simulink model "CH3_1"  (Simulink 5.0)
settings: Solver=ode15s  SolverMode=SingleTasking  StartTime=0.0  StopTime=3/60  RelTol=1e-3  AbsTol=1e-3
libraries: powerlib_extras x3
Description:
  | 高苑科技大學 電機系
  | 電力電子實驗室
settings Model: Creator=徐瑞隆老師  LastModifiedBy=ELECTRONIC  ExtModeTrigMode=oneshot  ExtModeArmWhenConnect=off  MaxOrder=4  LimitDataPoints=off  BlockReductionOpt=off  BooleanDataType=off  RTWTemplateMakefile=grt_unix.tmf

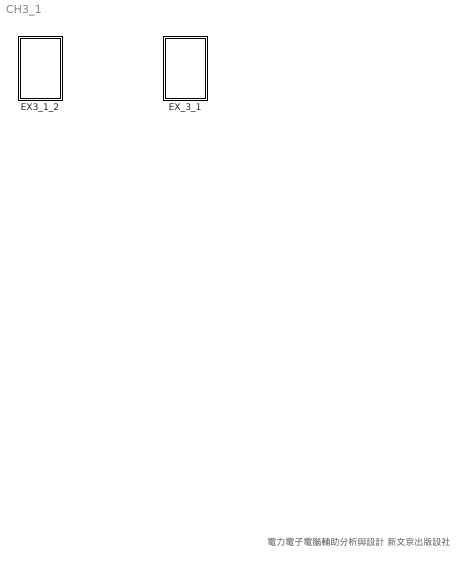
== system CH3_1 ==
  note: 電力電子電腦輔助分析與設計 新文京出版設社
  EX3_1_2 : Subsystem
  EX_3_1 : Subsystem

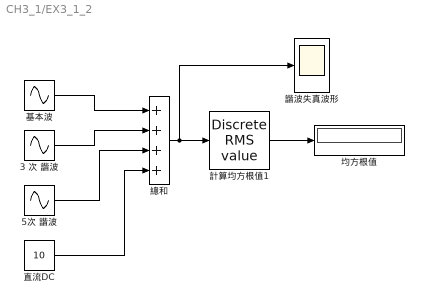
== system CH3_1/EX3_1_2 ==
  "3 次 諧波 " : Sin  Amplitude=8  Frequency=2*pi*180  Phase=1  SampleTime=0
  5次 諧波 : Sin  Amplitude=2  Frequency=2*pi*300  SampleTime=0
  "均方根值 " : Display
  直流DC : Constant  Value=10
  計算均方根值1 : powerlib_extras/Discrete Measurements/Discrete  RMS value  Freq=60  Mag_Init=0  Ts=50e-6
  基本波 : Sin  Amplitude=8  Frequency=2*pi*60  SampleTime=0
  諧波失真波形 : Scope
      settings: TimeRange=0.1  YMin=-3.5  YMax=3.5  SaveName=psb1phPWM3_str1  MaxDataPoints=50000
  總和 : Sum  Inputs=++++  SaturateOnIntegerOverflow=on  InputSameDT=on
  wires:
  直流DC/1 -> 總和/4
  總和/1 -> 計算均方根值1/1, 諧波失真波形/1
  5次 諧波/1 -> 總和/3
  "3 次 諧波 "/1 -> 總和/2
  基本波/1 -> 總和/1
  計算均方根值1/1 -> "均方根值 "/1

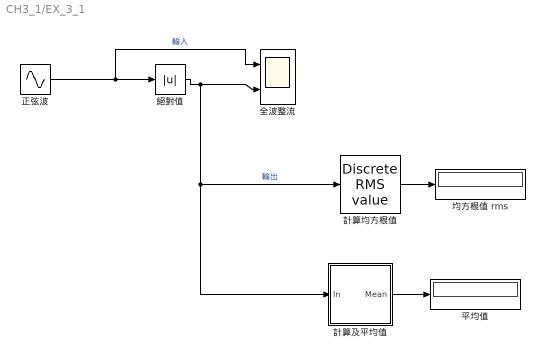
== system CH3_1/EX_3_1 ==
  平均值 : Display
  正弦波 : Sin  Amplitude=100  Frequency=2*pi*60  SampleTime=0
  全波整流 : Scope  NumInputPorts=2
      settings: TimeRange=0.05  YMin=0~-5  YMax=100~5  SaveName=psb1phPWM3_str  MaxDataPoints=50000
  均方根值 rms : Display
  "計算及平均值 " : Subsystem  AncestorBlock=|  mask(Discrete Mean value){Freq=60, Vinit=0, Ts=50e-6}
      | powerlib_extras/Discrete
      | Measurements/Discrete 
      | Mean value
      mask prompts: Freq "Fundamental frequency (Hz):"; Vinit "Initial input (DC component):"; Ts "Sample time:"
      mask help:
      | This block computes the mean value of the input signal over a running window of one cycle of the specified fundamental frequency.
      | For the first cycle of simulation, the ouput is held constant to the value specified by the parameter "Initial input".
      mask init:
      | SamplesPerCycle=1/Freq/Ts;
      | RoundSamplesPerCycle=ceil(SamplesPerCycle);
      | Delay=RoundSamplesPerCycle*Ts;
      | Corr1=(SamplesPerCycle-RoundSamplesPerCycle)/2;
      | Corr2=(SamplesPerCycle-RoundSamplesPerCycle)/SamplesPerCycle;
      | K1=Corr1*Corr2;
      | K2=Corr2 + Corr1*Corr2;
  計算均方根值 : powerlib_extras/Discrete Measurements/Discrete  RMS value  Freq=60  Mag_Init=0  Ts=50e-6
  絕對值 : Abs  SaturateOnIntegerOverflow=on
  wires:
  計算均方根值/1 -> 均方根值 rms/1
  正弦波/1 -> 絕對值/1, 全波整流/1  "輸入"
  絕對值/1 -> 計算均方根值/1, "計算及平均值 "/1(In), 全波整流/2  "輸出"
  "計算及平均值 "/1(Mean) -> 平均值/1

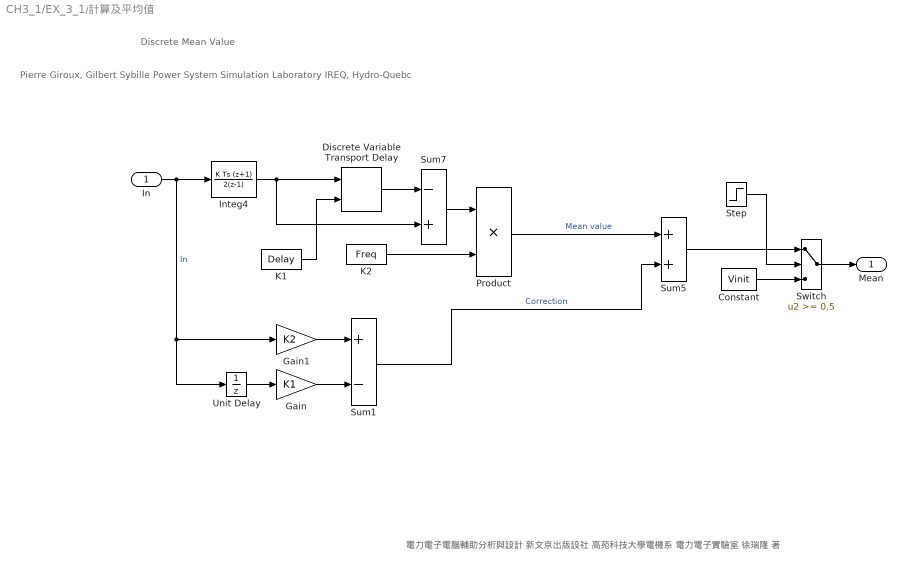
== system CH3_1/EX_3_1/計算及平均值  ==
  note: Pierre Giroux, Gilbert Sybille
      | Power System Simulation Laboratory
      | IREQ, Hydro-Quebc
  note: Discrete Mean Value
  note: 電力電子電腦輔助分析與設計  新文京出版設社
      | 高苑科技大學電機系
      | 電力電子實驗室
      | 徐瑞隆 著
  In : Inport
  Constant : Constant  Value=Vinit
  Discrete Variable Transport Delay : powerlib_extras/Discrete  Control Blocks/Discrete Variable Transport Delay  MaxDelay=Delay+Ts  InitialValue=0  Ts=Ts
  Gain : Gain  Gain=K1  SaturateOnIntegerOverflow=on
  Gain1 : Gain  Gain=K2  SaturateOnIntegerOverflow=on
  Integ4 : DiscreteIntegrator  IntegratorMethod=Trapezoidal  SampleTime=Ts
  K1 : Constant  Value=Delay
  K2 : Constant  Value=Freq
  Product : Product  SaturateOnIntegerOverflow=on  InputSameDT=on
  Step : Step  Time=1/Freq  SampleTime=Ts
  Sum1 : Sum  Inputs=+-  SaturateOnIntegerOverflow=on  InputSameDT=on
  Sum5 : Sum  SaturateOnIntegerOverflow=on  InputSameDT=on
  Sum7 : Sum  Inputs=-+  SaturateOnIntegerOverflow=on  InputSameDT=on
  Switch : Switch  Threshold=0.5  InputSameDT=on
  Unit Delay : UnitDelay  SampleTime=Ts
  Mean : Outport
  wires:
  Product/1 -> Sum5/1  "Mean value"
  Sum7/1 -> Product/1
  Integ4/1 -> Discrete Variable Transport Delay/1, Sum7/2
  K2/1 -> Product/2
  In/1 -> Integ4/1, Gain1/1, Unit Delay/1  "In"
  Sum5/1 -> Switch/1
  Step/1 -> Switch/2
  Constant/1 -> Switch/3
  Switch/1 -> Mean/1
  Discrete Variable Transport Delay/1 -> Sum7/1
  K1/1 -> Discrete Variable Transport Delay/2
  Gain1/1 -> Sum1/1
  Unit Delay/1 -> Gain/1
  Gain/1 -> Sum1/2
  Sum1/1 -> Sum5/2  "Correction"
